simulink model "Copy_of_simulator"  (R2024a)
settings: Solver=VariableStepAuto  StartTime=0.0  StopTime=50  RelTol=1e-3
values from neighbouring files (symbols this model uses):
  g = inputs(6,1)    [measFunction.m]    (also in stateFunction.m)
  k_f = 6.11e-8    (= 6.11e-08)    [Data.m]
  k_m = 1.5e-9    (= 1.5e-09)    [Data.m]
undefined symbols (not defined in the file or in its folder): A, B, C, L, m
libraries: slpidlib x7, simulink x2, shared6dof x1, sharedutil x1
(part 1 of 2)
settings Model: Creator=matteocolussi  LastModifiedBy=matteocolussi

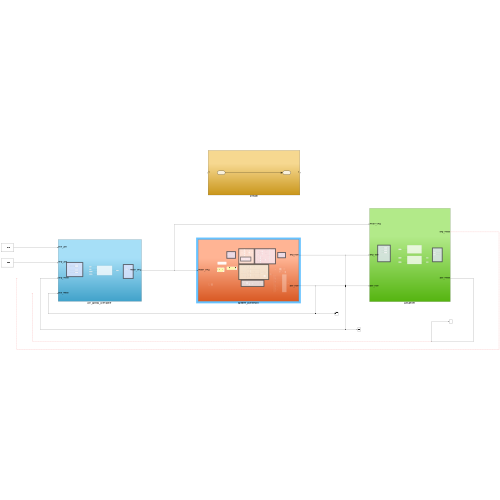
[thumbnail: Simulink's stored preview of the top-level diagram]
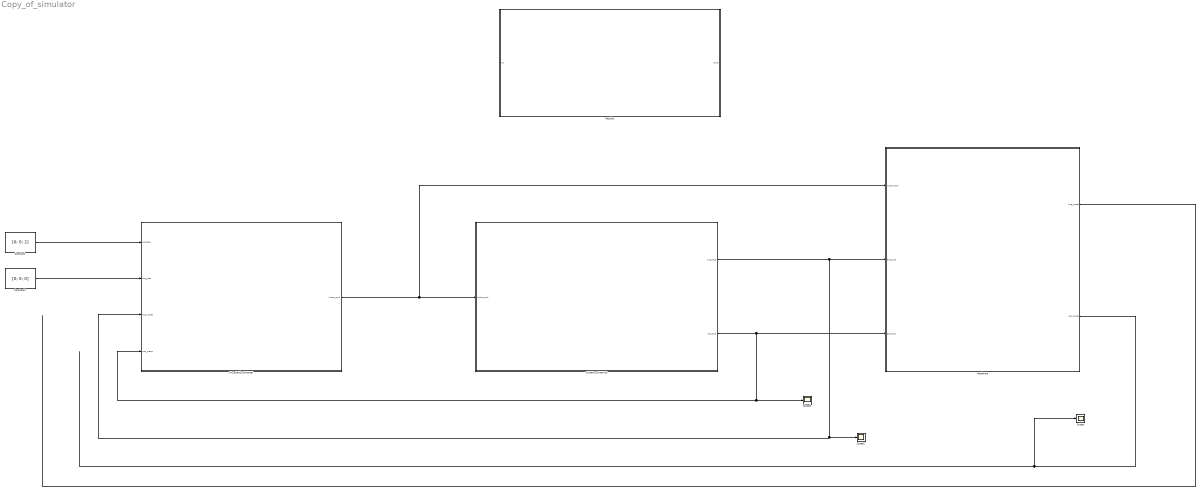
== system Copy_of_simulator ==
  Constant : Constant  Value=[0; 0; 2]
  Constant1 : Constant  Value=[0; 0; 0]
  Hardware : Subsystem
  On_Board_Computer : Subsystem
  Results : Subsystem
  Scope : Scope
  Scope1 : Scope
  Scope2 : Scope
  System_Dynamics : Subsystem
  wires:
  Constant1/1 -> On_Board_Computer/2(ang_des)
  On_Board_Computer/1(motor_cmd) -> Hardware/1(motor_cmd), System_Dynamics/1(motor_cmd)
  System_Dynamics/1(ang_true) -> Hardware/2(ang_true), On_Board_Computer/3(ang_meas), Scope2/1
  System_Dynamics/2(pos_true) -> Scope1/1, On_Board_Computer/4(pos_meas), Hardware/3(pos_true)
  Hardware/1(ang_meas) -> ?
  Hardware/2(pos_meas) -> Scope/1
  Constant/1 -> On_Board_Computer/1(pos_des)

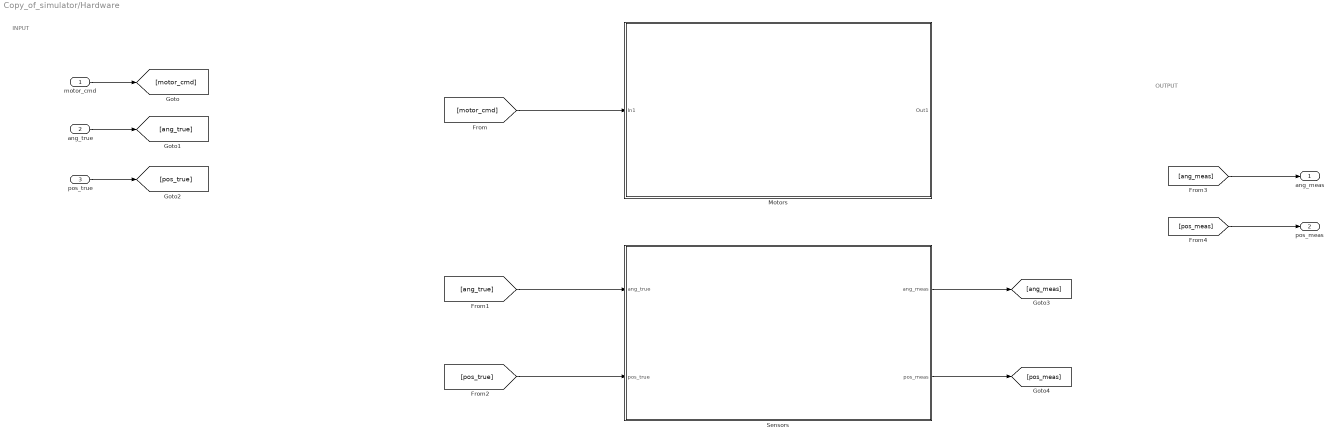
== system Copy_of_simulator/Hardware ==
  note: INPUT
  note: OUTPUT
  motor_cmd : Inport
  ang_true : Inport  Port=2
  pos_true : Inport  Port=3
  Motors : Subsystem
  Sensors : Subsystem
  ang_meas : Outport
  pos_meas : Outport  Port=2
  wires:
  motor_cmd/1 -> [motor_cmd]
  [motor_cmd] -> Motors/1(In1)
  ang_true/1 -> [ang_true]
  pos_true/1 -> [pos_true]
  [ang_true] -> Sensors/1(ang_true)
  [pos_true] -> Sensors/2(pos_true)
  Sensors/1(ang_meas) -> [ang_meas]
  Sensors/2(pos_meas) -> [pos_meas]
  [ang_meas] -> ang_meas/1
  [pos_meas] -> pos_meas/1

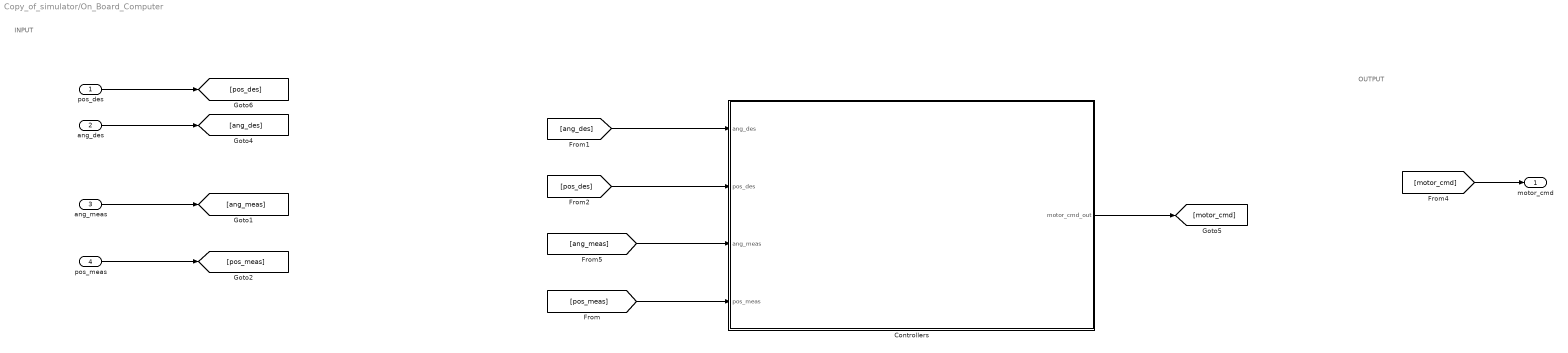
== system Copy_of_simulator/On_Board_Computer ==
  note: OUTPUT
  note: INPUT
  pos_des : Inport
  ang_des : Inport  Port=2
  ang_meas : Inport  Port=3
  pos_meas : Inport  Port=4
  Controllers : Subsystem
  motor_cmd : Outport
  wires:
  pos_des/1 -> [pos_des]
  [ang_des] -> Controllers/1(ang_des)
  [pos_des] -> Controllers/2(pos_des)
  ang_des/1 -> [ang_des]
  Controllers/1(motor_cmd_out) -> [motor_cmd]
  [motor_cmd] -> motor_cmd/1
  ang_meas/1 -> [ang_meas]
  pos_meas/1 -> [pos_meas]
  [pos_meas] -> Controllers/4(pos_meas)
  [ang_meas] -> Controllers/3(ang_meas)

== system Copy_of_simulator/Results ==
  In1 : Inport
  Out1 : Outport
  wires:
  In1/1 -> Out1/1

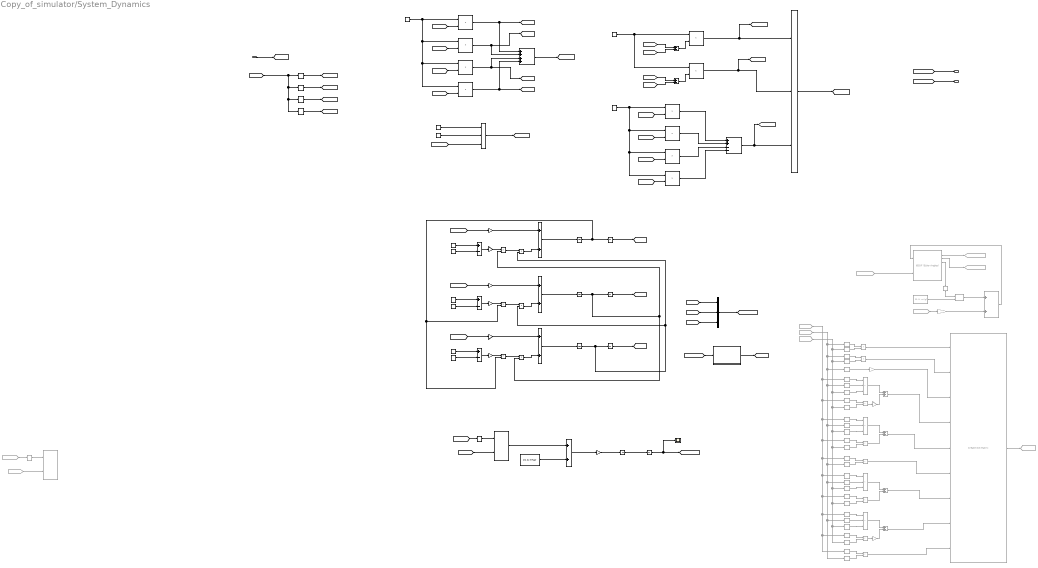
== system Copy_of_simulator/System_Dynamics ==
  note: ROTATIONAL DYNAMICS - EULER EQUATIONS
  note: FORCE VECTOR COMPUTATION
  note: Thrust computation
  note: INPUT
  note: Torque computation
  note: OUTPUT
  note: TRASLATIONAL DYNAMICS
  motor_cmd : Inport
  6DOF (Euler Angles) : shared6dof/6DOF (Euler Angles)  Commented=on  units=Metric (MKS)  mtype=Fixed  rep=Euler Angles  xme_0=[0 0 0]  Vm_0=[0 0 0]  eul_0=[0 0 0]  pm_0=[0 0 0]  mass_0=m  mass_e=0.5  mass_f=2.0  inertia=I  inertia_e=eye(3)  inertia_f=2*eye(3)  k_quat=1.0  vre_flag=on  abi_flag=on  aMode=0  xme_statename=''  Vm_statename=''  eul_statename=''  quat_statename=''  pm_statename=''  mass_statename=''
  Add{,1..4} (5 alike) : Sum  Inputs=+-
  Add{5,7..9} (4 alike) : Sum  Commented=on
  Add6 : Sum
  Constant : Constant  Value=k_f
  Constant1 : Constant  Value=k_m
  Constant10 : Constant  Value=A  VectorParams1D=off
  Constant11 : Constant  Value=B  VectorParams1D=off
  Constant13 : Constant  Value=[0, 0, m*g]'
  Constant14 : Constant  Commented=on  Value=[0; 0; -m*g]
  Constant2 : Constant  Value=L  VectorParams1D=off
  Constant3 : Constant  Value=0
  Constant4 : Constant  Value=0
  Constant5 : Constant  Value=C
  Constant6 : Constant  Value=B
  Constant7 : Constant  Value=C  VectorParams1D=off
  Constant9 : Constant  Value=A  VectorParams1D=off
  Cos{,1..4,6..8,12} (9 alike) : Trigonometry  Commented=on  Operator=cos
  Cos{5,9..11} (4 alike) : Trigonometry  Commented=on
  Create 3x3 Matrix : sharedutil/Create 3x3 Matrix  Commented=on  aMode=aMode
      settings: LibrarySourceBlock=aerolibutil/Create 3x3 Matrix
  From21 : From  Commented=on  GotoTag=F
  From23 : From  Commented=on  GotoTag=o_R_b
  From28 : From  Commented=on  GotoTag=F
  From29 : From  Commented=on  GotoTag=Mc
  From39 : From  Commented=on  GotoTag=phi_true
  From40 : From  Commented=on  GotoTag=theta_true
  From41 : From  Commented=on  GotoTag=psi_true
  Gain : Gain  Gain=1/A
  Gain1 : Gain  Gain=1/A
  Gain{6,8..10} (4 alike) : Gain  Commented=on  Gain=-1
  Gain2 : Gain  Gain=1/B
  Gain3 : Gain  Gain=1/B
  Gain4 : Gain  Gain=1/C
  Gain5 : Gain  Gain=1/C
  Gain7 : Gain  Gain=1/m
  Goto15 : Goto  Commented=on  GotoTag=o_R_b
  Goto29 : Goto  Commented=on  GotoTag=ang_true
  Goto30 : Goto  Commented=on  GotoTag=pos_true
  Integrator{6..11,18..19} (8 alike) : Integrator
  MATLAB Function : MATLAB Function  TreatAsAtomicUnit=on
  Matrix Multiply : Product  Commented=on  Multiplication=Matrix(*)
  Product{,1..9,11..16} (16 alike) : Product
  Product{10,19,21,23..24,26,28..29} (8 alike) : Product  Commented=on
  Product17 : Product  Commented=on  Multiplication=Matrix(*)
  Product18 : Product  Multiplication=Matrix(*)
  Product{20,22,25,27} (4 alike) : Product  Commented=on  Inputs=3
  Scope : Scope
  Selector : Selector  InputPortWidth=4  IndexOptions=Index vector (dialog)  Indices=1  OutputSizes=1
  Selector1 : Selector  InputPortWidth=4  IndexOptions=Index vector (dialog)  Indices=2  OutputSizes=1
  Selector2 : Selector  InputPortWidth=4  IndexOptions=Index vector (dialog)  Indices=3  OutputSizes=1
  Selector3 : Selector  InputPortWidth=4  IndexOptions=Index vector (dialog)  Indices=4  OutputSizes=1
  Sin{,1..6,8,10..11,13} (11 alike) : Trigonometry  Commented=on
  Sin{7,9,12,14..15} (5 alike) : Trigonometry  Commented=on  Operator=cos
  Sum : Sum  Inputs=++++
  Sum1 : Sum  Inputs=++--
  Sum2 : Sum
  Sum3 : Sum
  Sum4 : Sum
  Sum5 : Sum  Commented=on
  Transpose : Math  Commented=on  Operator=transpose
  Transpose1 : Math  Operator=transpose
  Transpose2 : Math  Commented=on  Operator=transpose
  Vector Concatenate : Concatenate  NumInputs=3
  Vector Concatenate1 : Concatenate  NumInputs=3
  Vector Concatenate3 : Concatenate  NumInputs=3
  ang_true : Outport
  pos_true : Outport  Port=2
  wires:
  motor_cmd/1 -> [motor_cmd]
  Selector/1 -> [w1_cmd]
  Selector1/1 -> [w2_cmd]
  Selector2/1 -> [w3_cmd]
  [motor_cmd] -> Selector3/1, Selector2/1, Selector1/1, Selector/1
  Selector3/1 -> [w4_cmd]
  Constant/1 -> Product3/1, Product2/1, Product1/1, Product/1
  [w1_cmd] -> Product/2
  [w2_cmd] -> Product1/2
  [w3_cmd] -> Product2/2
  [w4_cmd] -> Product3/2
  Product/1 -> [T1], Sum/1  "T1"
  Product1/1 -> Sum/2, [T2]  "T2"
  Product2/1 -> [T3], Sum/3  "T3"
  Product3/1 -> [T4], Sum/4  "T4"
  Sum/1 -> [T_tot]  "Thrust"
  [w2_cmd] -> Product5/2
  Constant1/1 -> Product7/1, Product6/1, Product5/1, Product4/1
  Product5/1 -> Sum1/2  "C2"
  Product6/1 -> Sum1/3  "C3"
  Product7/1 -> Sum1/4  "C4"
  [w1_cmd] -> Product4/2
  [w3_cmd] -> Product6/2
  Product4/1 -> Sum1/1  "C1"
  [w4_cmd] -> Product7/2
  Sum1/1 -> [Mc_zbody], Vector Concatenate/3  "Mc_zbody"
  Constant2/1 -> Product9/1, Product8/1
  [T3] -> Add/1
  [T4] -> Add/2
  Add/1 -> Product8/2
  [T2] -> Add1/1
  [T1] -> Add1/2
  Add1/1 -> Product9/2
  Product9/1 -> [Mc_ybody], Vector Concatenate/2  "Mc_ybody"
  Product8/1 -> [Mc_xbody], Vector Concatenate/1  "Mc_xbody"
  Vector Concatenate/1 -> [Mc]
  [T_tot] -> Vector Concatenate1/3
  Constant3/1 -> Vector Concatenate1/2
  Constant4/1 -> Vector Concatenate1/1
  Vector Concatenate1/1 -> [F]  "Force"
  [Mc_xbody] -> Gain1/1
  Constant6/1 -> Add2/1
  Add2/1 -> Gain/1
  Constant7/1 -> Add2/2
  Sum2/1 -> Integrator6/1  "phi_dotdot"
  Integrator7/1 -> [phi_true]  "phi"
  Gain/1 -> Product11/1
  Product11/1 -> Product12/1
  Product12/1 -> Sum2/2
  Gain1/1 -> Sum2/1
  Integrator9/1 -> [theta_true]  "theta"
  Gain3/1 -> Sum3/1
  Product14/1 -> Sum3/2
  [Mc_ybody] -> Gain3/1
  Gain2/1 -> Product13/1
  Integrator8/1 -> Integrator9/1, Product16/2, Product11/2  "theta_dot"
  Sum3/1 -> Integrator8/1  "theta_dotdot"
  Constant5/1 -> Add3/1
  Product13/1 -> Product14/1
  Add3/1 -> Gain2/1
  Constant9/1 -> Add3/2
  Integrator6/1 -> Integrator7/1, Product13/2, Product15/2  "phi_dot"
  Constant11/1 -> Add4/2
  Add4/1 -> Gain4/1
  Gain5/1 -> Sum4/1
  Constant10/1 -> Add4/1
  Gain4/1 -> Product15/1
  Integrator11/1 -> [psi_true]  "psi"
  Product16/1 -> Sum4/2
  [Mc_zbody] -> Gain5/1
  Integrator10/1 -> Product14/2, Product12/2, Integrator11/1  "psi_dot"
  Product15/1 -> Product16/1
  Sum4/1 -> Integrator10/1  "psi_dotdot"
  Vector Concatenate3/1 -> [ang_true]
  [theta_true] -> Vector Concatenate3/2
  [psi_true] -> Vector Concatenate3/3
  [phi_true] -> Vector Concatenate3/1
  From21/1 -> Transpose/1
  [ang_true] -> MATLAB Function/1(ang)
  MATLAB Function/1(o_R_b) -> [o_R_b]
  From23/1 -> Product17/2
  [ang_true] -> ang_true/1
  [pos_true] -> pos_true/1
  Transpose/1 -> Product17/1
  [F] -> Transpose1/1
  Add6/1 -> Gain7/1
  Transpose1/1 -> Product18/1
  Product18/1 -> Add6/1
  Gain7/1 -> Integrator18/1  "r_dotdot"
  [o_R_b] -> Product18/2
  Constant13/1 -> Add6/2
  Integrator18/1 -> Integrator19/1  "r_dot"
  Integrator19/1 -> [pos_true], Scope/1  "r"
  From29/1 -> 6DOF (Euler Angles)/2
  6DOF (Euler Angles)/3 -> Goto29/1
  6DOF (Euler Angles)/2 -> Goto30/1
  Constant14/1 -> Matrix Multiply/2
  6DOF (Euler Angles)/4 -> Transpose2/1
  From28/1 -> Gain8/1
  Matrix Multiply/1 -> Sum5/1
  Sum5/1 -> 6DOF (Euler Angles)/1
  Transpose2/1 -> Matrix Multiply/1
  Gain8/1 -> Sum5/2
  Cos/1 -> Product10/1
  Cos1/1 -> Product10/2
  Product10/1 -> Create 3x3 Matrix/1
  Product19/1 -> Create 3x3 Matrix/2
  Sin/1 -> Product19/2
  Cos2/1 -> Product19/1
  Sin1/1 -> Gain6/1
  Gain6/1 -> Create 3x3 Matrix/3
  Sin2/1 -> Product20/1
  Sin3/1 -> Product20/2
  Cos3/1 -> Product20/3
  Cos4/1 -> Product21/1
  Sin4/1 -> Product21/2
  Product20/1 -> Add5/1
  Product21/1 -> Gain9/1
  Gain9/1 -> Add5/2
  Add5/1 -> Create 3x3 Matrix/4
  Cos5/1 -> Product22/3
  Product22/1 -> Add7/1
  Add7/1 -> Create 3x3 Matrix/5
  Sin6/1 -> Product22/2
  Sin7/1 -> Product23/2
  Product23/1 -> Add7/2
  Sin5/1 -> Product22/1
  Cos6/1 -> Product23/1
  Sin8/1 -> Product24/1
  Cos7/1 -> Product24/2
  Product24/1 -> Create 3x3 Matrix/6
  Cos8/1 -> Product25/3
  Product25/1 -> Add8/1
  Sin11/1 -> Product26/2
  Add8/1 -> Create 3x3 Matrix/7
  Sin10/1 -> Product25/2
  Product26/1 -> Add8/2
  Sin9/1 -> Product25/1
  Cos9/1 -> Product26/1
  Product28/1 -> Gain10/1
  Cos10/1 -> Product27/3
  Product27/1 -> Add9/1
  Sin14/1 -> Product28/2
  Add9/1 -> Create 3x3 Matrix/8
  Sin13/1 -> Product27/2
  Gain10/1 -> Add9/2
  Sin12/1 -> Product27/1
  From41/1 -> Sin4/1, Cos5/1, Sin14/1, Cos10/1, Sin11/1, Cos8/1, Sin7/1, Cos3/1, Sin/1, Cos1/1
  Cos11/1 -> Product28/1
  Product29/1 -> Create 3x3 Matrix/9
  Sin15/1 -> Product29/2
  From39/1 -> Cos12/1, Cos11/1, Sin12/1, Cos9/1, Sin9/1, Sin8/1, Cos6/1, Sin5/1, Cos4/1, Sin2/1
  From40/1 -> Sin10/1, Sin15/1, Sin13/1, Cos7/1, Sin6/1, Sin3/1, Sin1/1, Cos2/1, Cos/1
  Cos12/1 -> Product29/1
  Create 3x3 Matrix/1 -> Goto15/1

== system Copy_of_simulator/Hardware/Motors ==
  In1 : Inport
  Out1 : Outport
  wires:
  In1/1 -> Out1/1

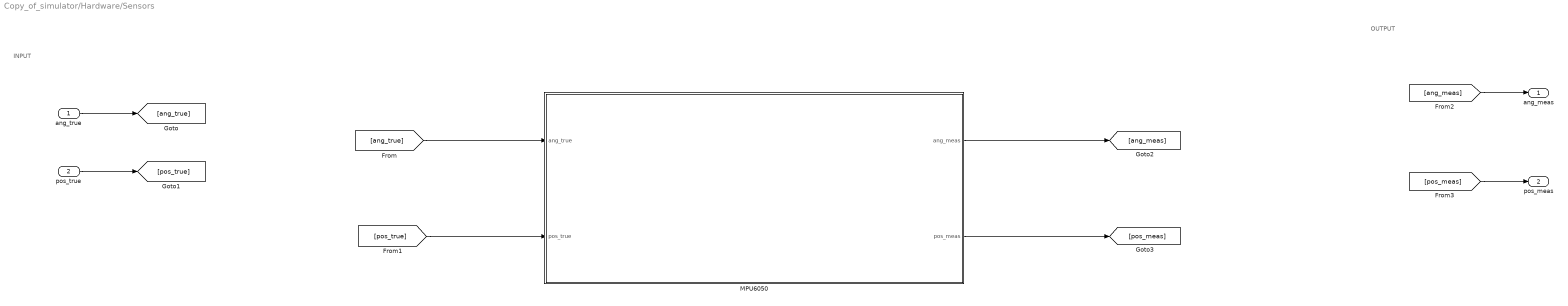
== system Copy_of_simulator/Hardware/Sensors ==
  note: OUTPUT
  note: INPUT
  ang_true : Inport
  pos_true : Inport  Port=2
  MPU6050 : Subsystem
  ang_meas : Outport
  pos_meas : Outport  Port=2
  wires:
  ang_true/1 -> [ang_true]
  pos_true/1 -> [pos_true]
  [ang_meas] -> ang_meas/1
  [pos_meas] -> pos_meas/1
  [ang_true] -> MPU6050/1(ang_true)
  [pos_true] -> MPU6050/2(pos_true)
  MPU6050/1(ang_meas) -> [ang_meas]
  MPU6050/2(pos_meas) -> [pos_meas]

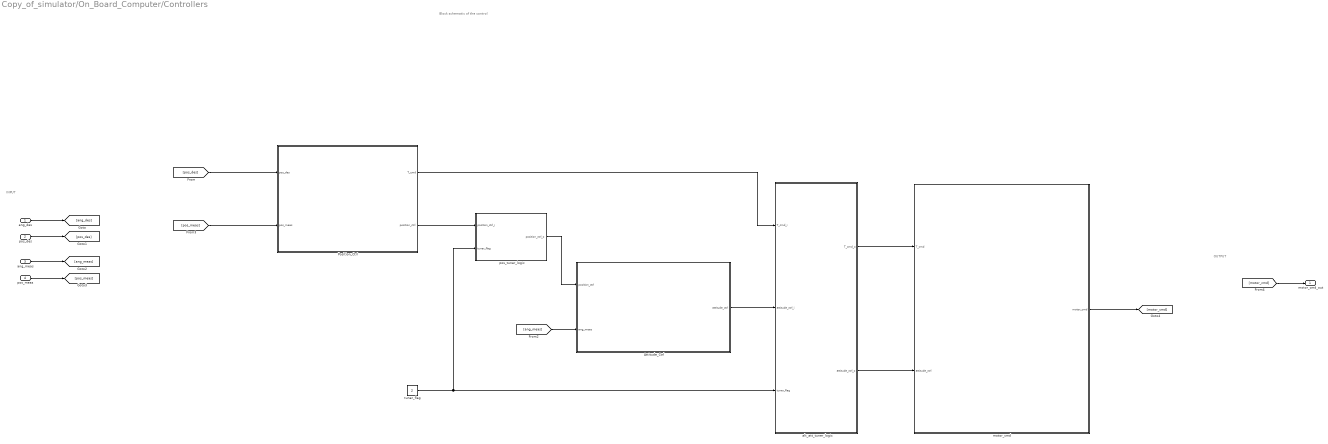
== system Copy_of_simulator/On_Board_Computer/Controllers ==
  note: Block schematic of the control
  note: OUTPUT
  note: INPUT
  ang_des : Inport
  pos_des : Inport  Port=2
  ang_meas : Inport  Port=3
  pos_meas : Inport  Port=4
  Attitude_Ctrl : Subsystem
  Position_Ctrl : Subsystem
  alt_att_tuner_logic : Subsystem
  motor_cmd : Subsystem
  pos_tuner_logic : Subsystem
  tuner_flag : Constant  Value=2
  motor_cmd_out : Outport
  wires:
  ang_des/1 -> [ang_des]
  pos_des/1 -> [pos_des]
  pos_meas/1 -> [pos_meas]
  ang_meas/1 -> [ang_meas]
  [ang_meas] -> Attitude_Ctrl/2(ang_meas)
  motor_cmd/1(motor_cmd) -> [motor_cmd]
  [motor_cmd] -> motor_cmd_out/1
  [pos_meas] -> Position_Ctrl/2(pos_meas)
  Attitude_Ctrl/1(attitude_ctrl) -> alt_att_tuner_logic/2(attitude_ctrl_i)
  tuner_flag/1 -> alt_att_tuner_logic/3(tuner_flag), pos_tuner_logic/2(tuner_flag)
  [pos_des] -> Position_Ctrl/1(pos_des)
  Position_Ctrl/2(position_ctrl) -> pos_tuner_logic/1(position_ctrl_i)
  pos_tuner_logic/1(position_ctrl_o) -> Attitude_Ctrl/1(position_ctrl)
  Position_Ctrl/1(T_cmd) -> alt_att_tuner_logic/1(T_cmd_i)
  alt_att_tuner_logic/1(T_cmd_o) -> motor_cmd/1(T_cmd)
  alt_att_tuner_logic/2(attitude_ctrl_o) -> motor_cmd/2(attitude_ctrl)

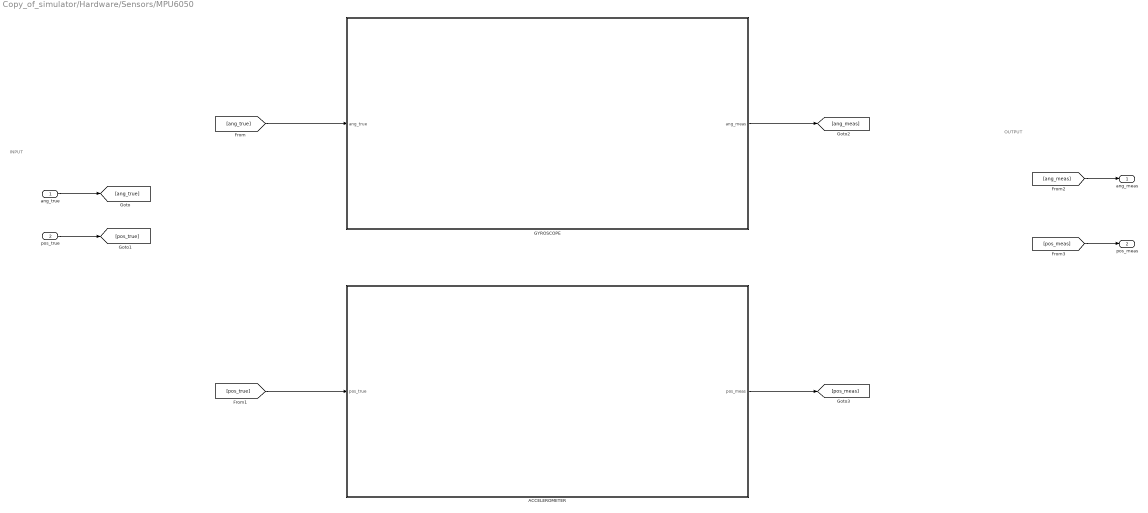
== system Copy_of_simulator/Hardware/Sensors/MPU6050 ==
  note: INPUT
  note: OUTPUT
  ang_true : Inport
  pos_true : Inport  Port=2
  ACCELEROMETER : Subsystem
  GYROSCOPE : Subsystem
  ang_meas : Outport
  pos_meas : Outport  Port=2
  wires:
  ang_true/1 -> [ang_true]
  pos_true/1 -> [pos_true]
  [pos_meas] -> pos_meas/1
  [ang_meas] -> ang_meas/1
  [ang_true] -> GYROSCOPE/1(ang_true)
  [pos_true] -> ACCELEROMETER/1(pos_true)
  GYROSCOPE/1(ang_meas) -> [ang_meas]
  ACCELEROMETER/1(pos_meas) -> [pos_meas]

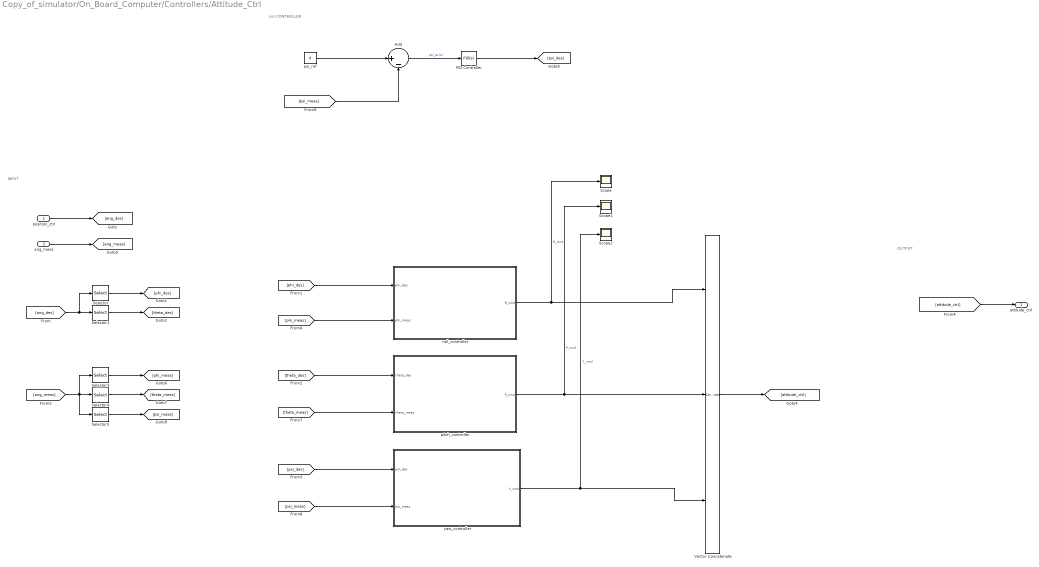
== system Copy_of_simulator/On_Board_Computer/Controllers/Attitude_Ctrl ==
  note: OUTPUT
  note: INPUT
  note: psi CONTROLLER
  position_ctrl : Inport
  ang_meas : Inport  Port=2
  Add : Sum  Inputs=|+-
  PID Controller : slpidlib/PID Controller  Controller=PID  Form=Parallel  TimeDomain=Continuous-time  UseExternalTs=off  SampleTime=-1  IntegratorMethod=Forward Euler  FilterMethod=Forward Euler  ControllerParametersSource=internal  P=1  I=0.8  UseKiTs=off  D=0.2  UseExternalDerivativeSource=off  N=100  UseFilter=on  TunerSelectOption=Transfer Function Based (PID Tuner App)  InitialConditionSource=internal  InitialConditionForIntegrator=0  InitialConditionForFilter=0  DifferentiatorICPrevScaledInput=0  ExternalReset=none  TrackingMode=off  Kt=1  LimitOutput=off  SatLimitsSource=internal  UpperSaturationLimit=inf  LowerSaturationLimit=-inf  LinearizeAsGain=on  AntiWindupMode=none  Kb=1  LimitIntegrator=off  UpperIntegratorSaturationLimit=inf  LowerIntegratorSaturationLimit=-inf  POutMin=[]  POutMax=[]  IOutMin=[]  IOutMax=[]  DOutMin=[]  DOutMax=[]  NOutMin=[]  NOutMax=[]  SumOutMin=[]  SumOutMax=[]  SaturationOutMin=[]  SaturationOutMax=[]  PParamMin=[]  PParamMax=[]  IParamMin=[]  IParamMax=[]  DParamMin=[]  DParamMax=[]  NParamMin=[]  NParamMax=[]  KbParamMin=[]  KbParamMax=[]  KtParamMin=[]  KtParamMax=[]  KbOutMin=[]  KbOutMax=[]  KtOutMin=[]  KtOutMax=[]  IntegratorOutMin=[]  IntegratorOutMax=[]  FilterOutMin=[]  FilterOutMax=[]  SumI1OutMin=[]  SumI1OutMax=[]  SumI2OutMin=[]  SumI2OutMax=[]  SumI3OutMin=[]  SumI3OutMax=[]  SumI4OutMin=[]  SumI4OutMax=[]  SumDOutMin=[]  SumDOutMax=[]  DifferentiatorOutMin=[]  DifferentiatorOutMax=[]  FilterDiffOutCoefMin=[]  FilterDiffOutCoefMax=[]  ReciprocalOutMin=[]  ReciprocalOutMax=[]  SumDenOutMin=[]  SumDenOutMax=[]  SumNumOutMin=[]  SumNumOutMax=[]  DivideOutMin=[]  DivideOutMax=[]  UdiffTsProdOutMin=[]  UdiffTsProdOutMax=[]  NTsProdOutMin=[]  NTsProdOutMax=[]  UintegralTsProdOutMin=[]  UintegralTsProdOutMax=[]  UngainTsProdOutMin=[]  UngainTsProdOutMax=[]  ClampingZeroOutDataTypeStr=Inherit: Inherit via back propagation  ClampingZeroOutMin=[]  ClampingZeroOutMax=[]  FilterDenConstantOutDataTypeStr=Inherit: Inherit via back propagation  FilterDenConstantOutMin=[]  FilterDenConstantOutMax=[]  PCopyOutDataTypeStr=Inherit: Inherit via back propagation  PCopyOutMin=[]  PCopyOutMax=[]  NCopyOutDataTypeStr=Inherit: Inherit via back propagation  NCopyOutMin=[]  NCopyOutMax=[]  IntegratorContinuousStateAttributes=''  IntegratorStateMustResolveToSignalObject=off  IntegratorRTWStateStorageClass=Auto  FilterContinuousStateAttributes=''  FilterStateMustResolveToSignalObject=off  FilterRTWStateStorageClass=Auto  ParallelPVariant=InternalParameters  IdealPVariant=Disabled  IVariant=InternalParameters  DVariant=InternalParameters  IntegratorVariant=Continuous  SatVariant=Disabled  AWVariant=Passthrough  PCopyVariant=Disabled  TRVariant=Disabled  FdbkBlocksVariant=Forward  IdealPFdbkVariant=Disabled  SatFdbkVariant=Disabled  DerivativeFilterVariant=ContFilter  NVariant=InternalParameters  NCopyVariant=Disabled  FilterICVariant=InternalICsFilter  IntegratorICVariant=InternalICs  ExternalResetVariant=Disabled  TRSumVariant=Passthrough  SumFdbkVariant=Disabled  SumVariant=Sum_PID  TsampFilterVariant=InternalTs  TsampNgainVariant=Passthrough  TsampIntegralVariant=Disabled_SignalSpec  ExternalSaturationOutDataTypeStr=Inherit: Same as second input  DerivativeSourceVariant=ErrorSignal
  Scope : Scope
  Scope1 : Scope
  Scope2 : Scope
  Selector : Selector  InputPortWidth=2  IndexOptions=Index vector (dialog)  Indices=1  OutputSizes=1
  Selector1 : Selector  InputPortWidth=2  IndexOptions=Index vector (dialog)  Indices=2  OutputSizes=1
  Selector3 : Selector  InputPortWidth=3  IndexOptions=Index vector (dialog)  Indices=1  OutputSizes=1
  Selector4 : Selector  InputPortWidth=3  IndexOptions=Index vector (dialog)  Indices=2  OutputSizes=1
  Selector5 : Selector  InputPortWidth=3  IndexOptions=Index vector (dialog)  Indices=3  OutputSizes=1
  Vector Concatenate : Concatenate  NumInputs=3
  pitch_controller : Subsystem
  psi_ref : Constant  Value=0
  roll_controller : Subsystem
  yaw_controller : Subsystem
  attitude_ctrl : Outport
  wires:
  position_ctrl/1 -> [ang_des]
  [phi_des] -> roll_controller/1(phi_des)
  [theta_des] -> pitch_controller/1(theta_des)
  [psi_des] -> yaw_controller/1(psi_des)
  roll_controller/1(R_cmd) -> Vector Concatenate/1, Scope/1  "R_cmd"
  pitch_controller/1(P_cmd) -> Scope1/1, Vector Concatenate/2  "P_cmd"
  yaw_controller/1(Y_cmd) -> Scope2/1, Vector Concatenate/3  "Y_cmd"
  ang_meas/1 -> [ang_meas]
  [phi_meas] -> roll_controller/2(phi_meas)
  [theta_meas] -> pitch_controller/2(theta_meas)
  [psi_meas] -> yaw_controller/2(psi_meas)
  Selector/1 -> [phi_des]
  [ang_des] -> Selector1/1, Selector/1
  Selector1/1 -> [theta_des]
  [ang_meas] -> Selector5/1, Selector4/1, Selector3/1
  Selector4/1 -> [theta_meas]
  Selector5/1 -> [psi_meas]
  Selector3/1 -> [phi_meas]
  Vector Concatenate/1 -> [attitude_ctrl]
  [attitude_ctrl] -> attitude_ctrl/1
  psi_ref/1 -> Add/1
  Add/1 -> PID Controller/1  "psi_error"
  PID Controller/1 -> [psi_des]
  [psi_meas] -> Add/2

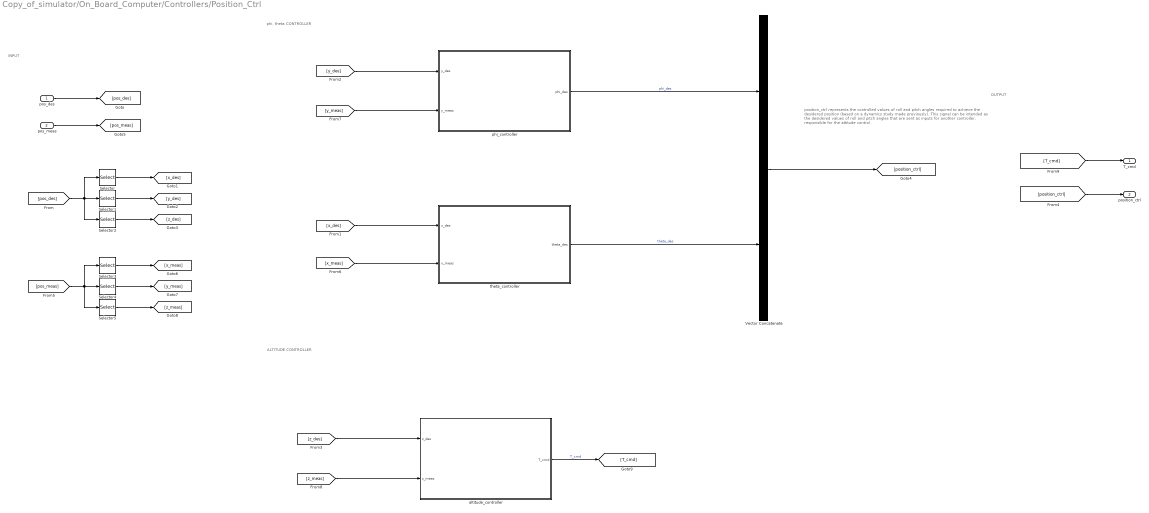
== system Copy_of_simulator/On_Board_Computer/Controllers/Position_Ctrl ==
  note: position_ctrl represents the controlled values of roll and pitch angles required to achieve the desidered position (based on a dynamics study made previously).
      |
      | This signal can be intended as the desidered values of roll and pitch angles that are sent as inputs for another controller, responsible for the attitude control .
  note: ALTITUDE CONTROLLER
  note: phi, theta CONTROLLER
  note: INPUT
  note: OUTPUT
  pos_des : Inport
  pos_meas : Inport  Port=2
  Selector : Selector  InputPortWidth=3  IndexOptions=Index vector (dialog)  Indices=1  OutputSizes=1
  Selector1 : Selector  InputPortWidth=3  IndexOptions=Index vector (dialog)  Indices=2  OutputSizes=1
  Selector2 : Selector  InputPortWidth=3  IndexOptions=Index vector (dialog)  Indices=3  OutputSizes=1
  Selector3 : Selector  InputPortWidth=3  IndexOptions=Index vector (dialog)  Indices=1  OutputSizes=1
  Selector4 : Selector  InputPortWidth=3  IndexOptions=Index vector (dialog)  Indices=2  OutputSizes=1
  Selector5 : Selector  InputPortWidth=3  IndexOptions=Index vector (dialog)  Indices=3  OutputSizes=1
  Vector Concatenate : Concatenate
  altitude_controller : Subsystem
  phi_controller : Subsystem
  theta_controller : Subsystem
  T_cmd : Outport
  position_ctrl : Outport  Port=2
  wires:
  Selector3/1 -> [x_meas]
  Selector4/1 -> [y_meas]
  [pos_meas] -> Selector5/1, Selector4/1, Selector3/1
  pos_meas/1 -> [pos_meas]
  Selector5/1 -> [z_meas]
  [pos_des] -> Selector2/1, Selector1/1, Selector/1
  Selector/1 -> [x_des]
  pos_des/1 -> [pos_des]
  Selector1/1 -> [y_des]
  Selector2/1 -> [z_des]
  [y_meas] -> phi_controller/2(y_meas)
  [x_des] -> theta_controller/1(x_des)
  [y_des] -> phi_controller/1(y_des)
  [x_meas] -> theta_controller/2(x_meas)
  [position_ctrl] -> position_ctrl/1
  Vector Concatenate/1 -> [position_ctrl]
  theta_controller/1(theta_des) -> Vector Concatenate/2  "theta_des"
  [z_meas] -> altitude_controller/2(z_meas)
  [z_des] -> altitude_controller/1(z_des)
  altitude_controller/1(T_cmd) -> [T_cmd]  "T_cmd"
  [T_cmd] -> T_cmd/1
  phi_controller/1(phi_des) -> Vector Concatenate/1  "phi_des"

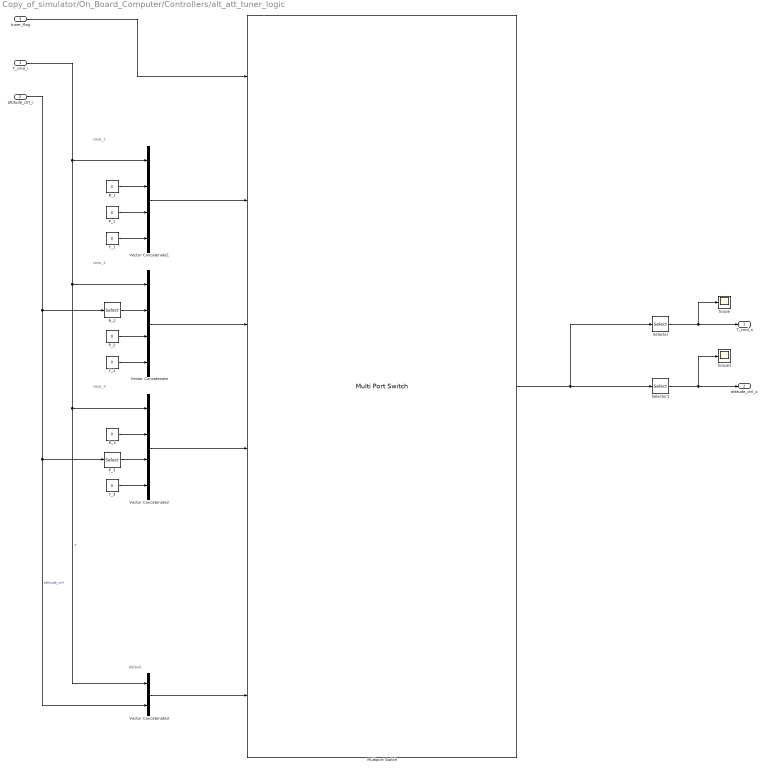
== system Copy_of_simulator/On_Board_Computer/Controllers/alt_att_tuner_logic ==
  note: case_2
  note: case_1
  note: case_3
  note: default
  T_cmd_i : Inport
  attitude_ctrl_i : Inport  Port=2
  tuner_flag : Inport  Port=3
  Multiport Switch : MultiPortSwitch  Inputs=5  SaturateOnIntegerOverflow=off  InputSameDT=off
  P_1 : Constant  Value=0
  P_2 : Constant  Value=0
  P_3 : Selector  InputPortWidth=3  IndexOptions=Index vector (dialog)  Indices=2  OutputSizes=1
  R_1 : Constant  Value=0
  R_2 : Selector  InputPortWidth=3  IndexOptions=Index vector (dialog)  Indices=1  OutputSizes=1
  R_3 : Constant  Value=0
  Scope : Scope
  Scope1 : Scope
  Selector : Selector  InputPortWidth=4  IndexOptions=Index vector (dialog)  Indices=1  OutputSizes=1
  Selector1 : Selector  InputPortWidth=4  IndexOptions=Index vector (dialog)  Indices=2:4  OutputSizes=1
  Vector Concatenate : Concatenate  NumInputs=4
  Vector Concatenate1 : Concatenate  NumInputs=4
  Vector Concatenate2 : Concatenate  NumInputs=4
  Vector Concatenate3 : Concatenate
  Y_1 : Constant  Value=0
  Y_2 : Constant  Value=0
  Y_3 : Constant  Value=0
  T_cmd_o : Outport
  attitude_ctrl_o : Outport  Port=2
  wires:
  tuner_flag/1 -> Multiport Switch/1
  Vector Concatenate/1 -> Multiport Switch/3
  P_2/1 -> Vector Concatenate/3
  Y_2/1 -> Vector Concatenate/4
  Multiport Switch/1 -> Selector/1, Selector1/1
  Selector/1 -> Scope/1, T_cmd_o/1
  Selector1/1 -> Scope1/1, attitude_ctrl_o/1
  R_2/1 -> Vector Concatenate/2
  R_1/1 -> Vector Concatenate1/2
  P_1/1 -> Vector Concatenate1/3
  Y_1/1 -> Vector Concatenate1/4
  Vector Concatenate1/1 -> Multiport Switch/2
  P_3/1 -> Vector Concatenate2/3
  Y_3/1 -> Vector Concatenate2/4
  Vector Concatenate2/1 -> Multiport Switch/4
  R_3/1 -> Vector Concatenate2/2
  T_cmd_i/1 -> Vector Concatenate3/1, Vector Concatenate2/1, Vector Concatenate/1, Vector Concatenate1/1  "T"
  Vector Concatenate3/1 -> Multiport Switch/6
  attitude_ctrl_i/1 -> Vector Concatenate3/2, P_3/1, R_2/1  "attitude_ctrl"

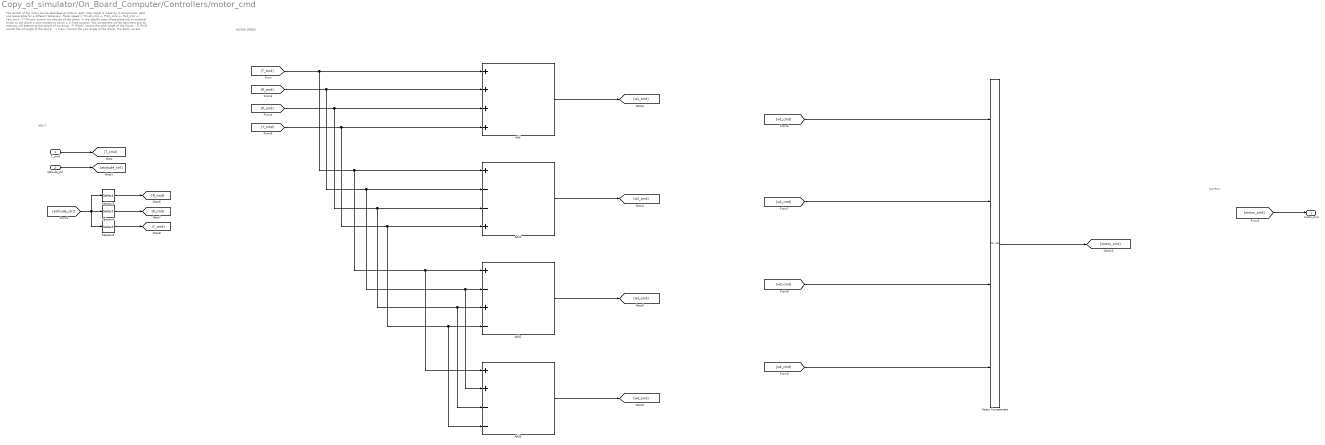
== system Copy_of_simulator/On_Board_Computer/Controllers/motor_cmd ==
  note: The control of the rotors can be described as follows:
      |
      | each rotor signal is made by 4 components, each one responsible for a different behaviour:
      |
      | Rotor speed = Thrust_cmd +- Pitch_cmd +- Roll_cmd +- Yaw_cmd
      |
      | - T (Thrust): control the altitude of the drone. In the specific case where there are no
      | external forces or the drone is commanded to hover in a fixed position,
      | this component will be dominant and its intensity will determine the height
      | of hovering;
      | - P (Pitch): control the pitch angle of the drone;
      | - R (Roll): control the roll angle of the drone;
      | - Y (Yaw): control the yaw angle of the drone;
      |
      | The block we are currently in is responsible for the computation of each component and their correct combination, which is different for every single rotor.
  note: MOTOR SPEED
  note: OUTPUT
  note: INPUT
  T_cmd : Inport
  attitude_ctrl : Inport  Port=2
  Add : Sum  Inputs=++++
  Add1 : Sum  Inputs=+--+
  Add2 : Sum  Inputs=+-+-
  Add3 : Sum  Inputs=++--
  Selector3 : Selector  InputPortWidth=3  IndexOptions=Index vector (dialog)  Indices=1  OutputSizes=1
  Selector4 : Selector  InputPortWidth=3  IndexOptions=Index vector (dialog)  Indices=2  OutputSizes=1
  Selector5 : Selector  InputPortWidth=3  IndexOptions=Index vector (dialog)  Indices=3  OutputSizes=1
  Vector Concatenate : Concatenate  NumInputs=4
  motor_cmd : Outport
  wires:
  T_cmd/1 -> [T_cmd]
  [motor_cmd] -> motor_cmd/1
  attitude_ctrl/1 -> [attitude_ctrl]
  Selector3/1 -> [R_cmd]
  Selector4/1 -> [P_cmd]
  [attitude_ctrl] -> Selector5/1, Selector4/1, Selector3/1
  Selector5/1 -> [Y_cmd]
  [T_cmd] -> Add/1, Add2/1, Add3/1, Add1/1
  [R_cmd] -> Add/2, Add3/2, Add2/2, Add1/2
  [P_cmd] -> Add/3, Add1/3, Add3/3, Add2/3
  [Y_cmd] -> Add/4, Add1/4, Add3/4, Add2/4
  Add/1 -> [w1_cmd]
  Add1/1 -> [w2_cmd]
  Add2/1 -> [w3_cmd]
  Add3/1 -> [w4_cmd]
  Vector Concatenate/1 -> [motor_cmd]
  [w2_cmd] -> Vector Concatenate/2
  [w1_cmd] -> Vector Concatenate/1
  [w3_cmd] -> Vector Concatenate/3
  [w4_cmd] -> Vector Concatenate/4

== system Copy_of_simulator/On_Board_Computer/Controllers/pos_tuner_logic ==
  note: case_2
  note: case_3
  position_ctrl_i : Inport
  tuner_flag : Inport  Port=2
  Multiport Switch : MultiPortSwitch  Inputs=5  SaturateOnIntegerOverflow=off  InputSameDT=off
  Scope : Scope
  Vector Concatenate : Concatenate
  Vector Concatenate1 : Concatenate
  phi_des_2 : Constant  Value=2
  phi_des_3 : Constant  Value=0
  theta_des_2 : Constant  Value=0
  theta_des_3 : Constant  Value=2
  position_ctrl_o : Outport
  wires:
  tuner_flag/1 -> Multiport Switch/1
  Multiport Switch/1 -> Scope/1, position_ctrl_o/1
  position_ctrl_i/1 -> Multiport Switch/6
  Vector Concatenate/1 -> Multiport Switch/3
  phi_des_2/1 -> Vector Concatenate/1
  theta_des_2/1 -> Vector Concatenate/2
  theta_des_3/1 -> Vector Concatenate1/2
  phi_des_3/1 -> Vector Concatenate1/1
  Vector Concatenate1/1 -> Multiport Switch/4

== system Copy_of_simulator/Hardware/Sensors/MPU6050/ACCELEROMETER ==
  pos_true : Inport
  Band-Limited White Noise : simulink/Sources/Band-Limited White Noise  Cov=[0.1]  Ts=0.1  seed=[23341]
  Sum : Sum  Inputs=|++
  pos_meas : Outport
  wires:
  Band-Limited White Noise/1 -> Sum/2
  pos_true/1 -> Sum/1
  Sum/1 -> pos_meas/1

== system Copy_of_simulator/Hardware/Sensors/MPU6050/GYROSCOPE ==
  ang_true : Inport
  Band-Limited White Noise : simulink/Sources/Band-Limited White Noise  Cov=[0.1]  Ts=0.1  seed=[23341]
  Sum : Sum  Inputs=|++
  ang_meas : Outport
  wires:
  ang_true/1 -> Sum/1
  Band-Limited White Noise/1 -> Sum/2
  Sum/1 -> ang_meas/1

== system Copy_of_simulator/On_Board_Computer/Controllers/Attitude_Ctrl/pitch_controller ==
  note: OUTPUT
  note: INPUT
  note: SENSOR DYNAMICS
      | TBD
  theta_des : Inport
  theta_meas : Inport  Port=2
  Add : Sum  Inputs=|+-
  PID Controller : slpidlib/PID Controller  Controller=PID  Form=Parallel  TimeDomain=Continuous-time  UseExternalTs=off  SampleTime=-1  IntegratorMethod=Forward Euler  FilterMethod=Forward Euler  ControllerParametersSource=internal  P=-17625.8547786025  I=-825.150483451763  UseKiTs=off  D=-92450.7642106306  UseExternalDerivativeSource=off  N=5.45397025421619  UseFilter=on  TunerSelectOption=Transfer Function Based (PID Tuner App)  InitialConditionSource=internal  InitialConditionForIntegrator=0  InitialConditionForFilter=0  DifferentiatorICPrevScaledInput=0  ExternalReset=none  TrackingMode=off  Kt=1  LimitOutput=off  SatLimitsSource=internal  UpperSaturationLimit=inf  LowerSaturationLimit=-inf  LinearizeAsGain=on  AntiWindupMode=none  Kb=1  LimitIntegrator=off  UpperIntegratorSaturationLimit=inf  LowerIntegratorSaturationLimit=-inf  POutMin=[]  POutMax=[]  IOutMin=[]  IOutMax=[]  DOutMin=[]  DOutMax=[]  NOutMin=[]  NOutMax=[]  SumOutMin=[]  SumOutMax=[]  SaturationOutMin=[]  SaturationOutMax=[]  PParamMin=[]  PParamMax=[]  IParamMin=[]  IParamMax=[]  DParamMin=[]  DParamMax=[]  NParamMin=[]  NParamMax=[]  KbParamMin=[]  KbParamMax=[]  KtParamMin=[]  KtParamMax=[]  KbOutMin=[]  KbOutMax=[]  KtOutMin=[]  KtOutMax=[]  IntegratorOutMin=[]  IntegratorOutMax=[]  FilterOutMin=[]  FilterOutMax=[]  SumI1OutMin=[]  SumI1OutMax=[]  SumI2OutMin=[]  SumI2OutMax=[]  SumI3OutMin=[]  SumI3OutMax=[]  SumI4OutMin=[]  SumI4OutMax=[]  SumDOutMin=[]  SumDOutMax=[]  DifferentiatorOutMin=[]  DifferentiatorOutMax=[]  FilterDiffOutCoefMin=[]  FilterDiffOutCoefMax=[]  ReciprocalOutMin=[]  ReciprocalOutMax=[]  SumDenOutMin=[]  SumDenOutMax=[]  SumNumOutMin=[]  SumNumOutMax=[]  DivideOutMin=[]  DivideOutMax=[]  UdiffTsProdOutMin=[]  UdiffTsProdOutMax=[]  NTsProdOutMin=[]  NTsProdOutMax=[]  UintegralTsProdOutMin=[]  UintegralTsProdOutMax=[]  UngainTsProdOutMin=[]  UngainTsProdOutMax=[]  ClampingZeroOutDataTypeStr=Inherit: Inherit via back propagation  ClampingZeroOutMin=[]  ClampingZeroOutMax=[]  FilterDenConstantOutDataTypeStr=Inherit: Inherit via back propagation  FilterDenConstantOutMin=[]  FilterDenConstantOutMax=[]  PCopyOutDataTypeStr=Inherit: Inherit via back propagation  PCopyOutMin=[]  PCopyOutMax=[]  NCopyOutDataTypeStr=Inherit: Inherit via back propagation  NCopyOutMin=[]  NCopyOutMax=[]  IntegratorContinuousStateAttributes=''  IntegratorStateMustResolveToSignalObject=off  IntegratorRTWStateStorageClass=Auto  FilterContinuousStateAttributes=''  FilterStateMustResolveToSignalObject=off  FilterRTWStateStorageClass=Auto  ParallelPVariant=InternalParameters  IdealPVariant=Disabled  IVariant=InternalParameters  DVariant=InternalParameters  IntegratorVariant=Continuous  SatVariant=Disabled  AWVariant=Passthrough  PCopyVariant=Disabled  TRVariant=Disabled  FdbkBlocksVariant=Forward  IdealPFdbkVariant=Disabled  SatFdbkVariant=Disabled  DerivativeFilterVariant=ContFilter  NVariant=InternalParameters  NCopyVariant=Disabled  FilterICVariant=InternalICsFilter  IntegratorICVariant=InternalICs  ExternalResetVariant=Disabled  TRSumVariant=Passthrough  SumFdbkVariant=Disabled  SumVariant=Sum_PID  TsampFilterVariant=InternalTs  TsampNgainVariant=Passthrough  TsampIntegralVariant=Disabled_SignalSpec  ExternalSaturationOutDataTypeStr=Inherit: Same as second input  DerivativeSourceVariant=ErrorSignal
  P_cmd : Outport
  wires:
  Add/1 -> PID Controller/1  "theta_error"
  [P_cmd] -> P_cmd/1
  [theta_des] -> Add/1
  theta_des/1 -> [theta_des]
  PID Controller/1 -> [P_cmd]
  theta_meas/1 -> [theta_meas]
  [theta_meas] -> Add/2

== system Copy_of_simulator/On_Board_Computer/Controllers/Attitude_Ctrl/roll_controller ==
  note: OUTPUT
  note: INPUT
  phi_des : Inport
  phi_meas : Inport  Port=2
  Add : Sum  Inputs=|+-
  PID Controller : slpidlib/PID Controller  Controller=PID  Form=Parallel  TimeDomain=Continuous-time  UseExternalTs=off  SampleTime=-1  IntegratorMethod=Forward Euler  FilterMethod=Forward Euler  ControllerParametersSource=internal  P=-17625.8547786025  I=-825.150483451763  UseKiTs=off  D=-92450.7642106305  UseExternalDerivativeSource=off  N=5.45397025421619  UseFilter=on  TunerSelectOption=Transfer Function Based (PID Tuner App)  InitialConditionSource=internal  InitialConditionForIntegrator=0  InitialConditionForFilter=0  DifferentiatorICPrevScaledInput=0  ExternalReset=none  TrackingMode=off  Kt=1  LimitOutput=off  SatLimitsSource=internal  UpperSaturationLimit=inf  LowerSaturationLimit=-inf  LinearizeAsGain=on  AntiWindupMode=none  Kb=1  LimitIntegrator=off  UpperIntegratorSaturationLimit=inf  LowerIntegratorSaturationLimit=-inf  POutMin=[]  POutMax=[]  IOutMin=[]  IOutMax=[]  DOutMin=[]  DOutMax=[]  NOutMin=[]  NOutMax=[]  SumOutMin=[]  SumOutMax=[]  SaturationOutMin=[]  SaturationOutMax=[]  PParamMin=[]  PParamMax=[]  IParamMin=[]  IParamMax=[]  DParamMin=[]  DParamMax=[]  NParamMin=[]  NParamMax=[]  KbParamMin=[]  KbParamMax=[]  KtParamMin=[]  KtParamMax=[]  KbOutMin=[]  KbOutMax=[]  KtOutMin=[]  KtOutMax=[]  IntegratorOutMin=[]  IntegratorOutMax=[]  FilterOutMin=[]  FilterOutMax=[]  SumI1OutMin=[]  SumI1OutMax=[]  SumI2OutMin=[]  SumI2OutMax=[]  SumI3OutMin=[]  SumI3OutMax=[]  SumI4OutMin=[]  SumI4OutMax=[]  SumDOutMin=[]  SumDOutMax=[]  DifferentiatorOutMin=[]  DifferentiatorOutMax=[]  FilterDiffOutCoefMin=[]  FilterDiffOutCoefMax=[]  ReciprocalOutMin=[]  ReciprocalOutMax=[]  SumDenOutMin=[]  SumDenOutMax=[]  SumNumOutMin=[]  SumNumOutMax=[]  DivideOutMin=[]  DivideOutMax=[]  UdiffTsProdOutMin=[]  UdiffTsProdOutMax=[]  NTsProdOutMin=[]  NTsProdOutMax=[]  UintegralTsProdOutMin=[]  UintegralTsProdOutMax=[]  UngainTsProdOutMin=[]  UngainTsProdOutMax=[]  ClampingZeroOutDataTypeStr=Inherit: Inherit via back propagation  ClampingZeroOutMin=[]  ClampingZeroOutMax=[]  FilterDenConstantOutDataTypeStr=Inherit: Inherit via back propagation  FilterDenConstantOutMin=[]  FilterDenConstantOutMax=[]  PCopyOutDataTypeStr=Inherit: Inherit via back propagation  PCopyOutMin=[]  PCopyOutMax=[]  NCopyOutDataTypeStr=Inherit: Inherit via back propagation  NCopyOutMin=[]  NCopyOutMax=[]  IntegratorContinuousStateAttributes=''  IntegratorStateMustResolveToSignalObject=off  IntegratorRTWStateStorageClass=Auto  FilterContinuousStateAttributes=''  FilterStateMustResolveToSignalObject=off  FilterRTWStateStorageClass=Auto  ParallelPVariant=InternalParameters  IdealPVariant=Disabled  IVariant=InternalParameters  DVariant=InternalParameters  IntegratorVariant=Continuous  SatVariant=Disabled  AWVariant=Passthrough  PCopyVariant=Disabled  TRVariant=Disabled  FdbkBlocksVariant=Forward  IdealPFdbkVariant=Disabled  SatFdbkVariant=Disabled  DerivativeFilterVariant=ContFilter  NVariant=InternalParameters  NCopyVariant=Disabled  FilterICVariant=InternalICsFilter  IntegratorICVariant=InternalICs  ExternalResetVariant=Disabled  TRSumVariant=Passthrough  SumFdbkVariant=Disabled  SumVariant=Sum_PID  TsampFilterVariant=InternalTs  TsampNgainVariant=Passthrough  TsampIntegralVariant=Disabled_SignalSpec  ExternalSaturationOutDataTypeStr=Inherit: Same as second input  DerivativeSourceVariant=ErrorSignal
  R_cmd : Outport
  wires:
  phi_des/1 -> [phi_des]
  [phi_des] -> Add/1
  [R_cmd] -> R_cmd/1
  phi_meas/1 -> [phi_meas]
  [phi_meas] -> Add/2
  Add/1 -> PID Controller/1  "phi_error"
  PID Controller/1 -> [R_cmd]

== system Copy_of_simulator/On_Board_Computer/Controllers/Attitude_Ctrl/yaw_controller ==
  note: OUTPUT
  note: INPUT
  note: SENSOR DYNAMICS
      | TBD
  psi_des : Inport
  psi_meas : Inport  Port=2
  Add : Sum  Inputs=|+-
  PID Controller : slpidlib/PID Controller  Controller=PID  Form=Parallel  TimeDomain=Continuous-time  UseExternalTs=off  SampleTime=-1  IntegratorMethod=Forward Euler  FilterMethod=Forward Euler  ControllerParametersSource=internal  P=-2.16227850344127  I=-3.82729714855674  UseKiTs=off  D=-0.0839125504621507  UseExternalDerivativeSource=off  N=10.1322259704898  UseFilter=on  TunerSelectOption=Transfer Function Based (PID Tuner App)  InitialConditionSource=internal  InitialConditionForIntegrator=0  InitialConditionForFilter=0  DifferentiatorICPrevScaledInput=0  ExternalReset=none  TrackingMode=off  Kt=1  LimitOutput=off  SatLimitsSource=internal  UpperSaturationLimit=inf  LowerSaturationLimit=-inf  LinearizeAsGain=on  AntiWindupMode=none  Kb=1  LimitIntegrator=off  UpperIntegratorSaturationLimit=inf  LowerIntegratorSaturationLimit=-inf  POutMin=[]  POutMax=[]  IOutMin=[]  IOutMax=[]  DOutMin=[]  DOutMax=[]  NOutMin=[]  NOutMax=[]  SumOutMin=[]  SumOutMax=[]  SaturationOutMin=[]  SaturationOutMax=[]  PParamMin=[]  PParamMax=[]  IParamMin=[]  IParamMax=[]  DParamMin=[]  DParamMax=[]  NParamMin=[]  NParamMax=[]  KbParamMin=[]  KbParamMax=[]  KtParamMin=[]  KtParamMax=[]  KbOutMin=[]  KbOutMax=[]  KtOutMin=[]  KtOutMax=[]  IntegratorOutMin=[]  IntegratorOutMax=[]  FilterOutMin=[]  FilterOutMax=[]  SumI1OutMin=[]  SumI1OutMax=[]  SumI2OutMin=[]  SumI2OutMax=[]  SumI3OutMin=[]  SumI3OutMax=[]  SumI4OutMin=[]  SumI4OutMax=[]  SumDOutMin=[]  SumDOutMax=[]  DifferentiatorOutMin=[]  DifferentiatorOutMax=[]  FilterDiffOutCoefMin=[]  FilterDiffOutCoefMax=[]  ReciprocalOutMin=[]  ReciprocalOutMax=[]  SumDenOutMin=[]  SumDenOutMax=[]  SumNumOutMin=[]  SumNumOutMax=[]  DivideOutMin=[]  DivideOutMax=[]  UdiffTsProdOutMin=[]  UdiffTsProdOutMax=[]  NTsProdOutMin=[]  NTsProdOutMax=[]  UintegralTsProdOutMin=[]  UintegralTsProdOutMax=[]  UngainTsProdOutMin=[]  UngainTsProdOutMax=[]  ClampingZeroOutDataTypeStr=Inherit: Inherit via back propagation  ClampingZeroOutMin=[]  ClampingZeroOutMax=[]  FilterDenConstantOutDataTypeStr=Inherit: Inherit via back propagation  FilterDenConstantOutMin=[]  FilterDenConstantOutMax=[]  PCopyOutDataTypeStr=Inherit: Inherit via back propagation  PCopyOutMin=[]  PCopyOutMax=[]  NCopyOutDataTypeStr=Inherit: Inherit via back propagation  NCopyOutMin=[]  NCopyOutMax=[]  IntegratorContinuousStateAttributes=''  IntegratorStateMustResolveToSignalObject=off  IntegratorRTWStateStorageClass=Auto  FilterContinuousStateAttributes=''  FilterStateMustResolveToSignalObject=off  FilterRTWStateStorageClass=Auto  ParallelPVariant=InternalParameters  IdealPVariant=Disabled  IVariant=InternalParameters  DVariant=InternalParameters  IntegratorVariant=Continuous  SatVariant=Disabled  AWVariant=Passthrough  PCopyVariant=Disabled  TRVariant=Disabled  FdbkBlocksVariant=Forward  IdealPFdbkVariant=Disabled  SatFdbkVariant=Disabled  DerivativeFilterVariant=ContFilter  NVariant=InternalParameters  NCopyVariant=Disabled  FilterICVariant=InternalICsFilter  IntegratorICVariant=InternalICs  ExternalResetVariant=Disabled  TRSumVariant=Passthrough  SumFdbkVariant=Disabled  SumVariant=Sum_PID  TsampFilterVariant=InternalTs  TsampNgainVariant=Passthrough  TsampIntegralVariant=Disabled_SignalSpec  ExternalSaturationOutDataTypeStr=Inherit: Same as second input  DerivativeSourceVariant=ErrorSignal
  Y_cmd : Outport
  wires:
  Add/1 -> PID Controller/1  "psi_error"
  [Y_cmd] -> Y_cmd/1
  [psi_des] -> Add/1
  psi_des/1 -> [psi_des]
  PID Controller/1 -> [Y_cmd]
  psi_meas/1 -> [psi_meas]
  [psi_meas] -> Add/2

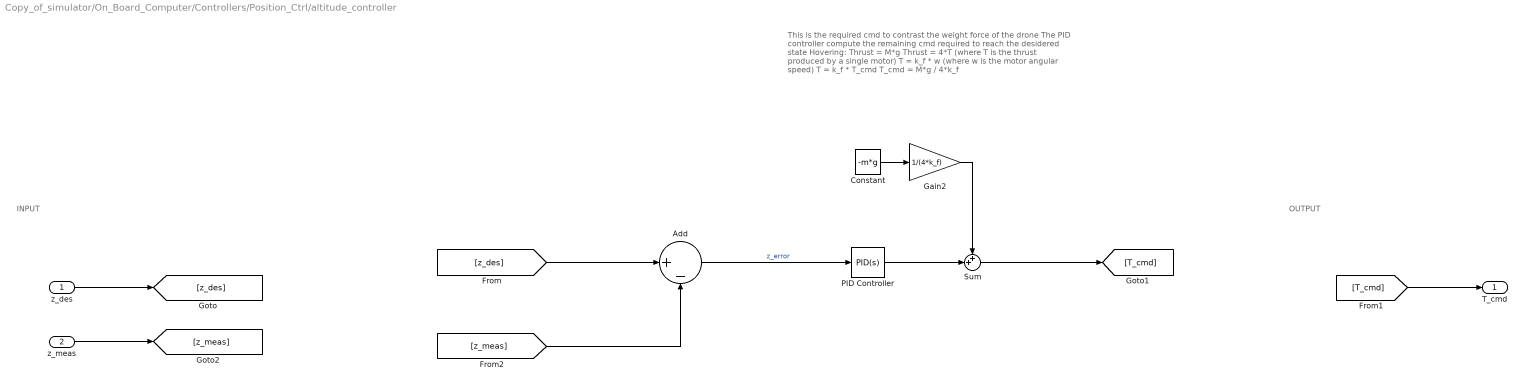
== system Copy_of_simulator/On_Board_Computer/Controllers/Position_Ctrl/altitude_controller ==
  note: OUTPUT
  note: INPUT
  note: This is the required cmd to contrast the weight force of the drone
      |
      | The PID controller compute the remaining cmd required to reach the
      | desidered state
      |
      | Hovering:
      | Thrust = M*g
      | Thrust = 4*T (where T is the thrust produced by a single motor)
      | T = k_f * w (where w is the motor angular speed)
      | T = k_f * T_cmd
      |
      | T_cmd = M*g / 4*k_f
  z_des : Inport
  z_meas : Inport  Port=2
  Add : Sum  Inputs=|+-
  Constant : Constant  Value=-m*g
  Gain2 : Gain  Gain=1/(4*k_f)
  PID Controller : slpidlib/PID Controller  Controller=PID  Form=Parallel  TimeDomain=Continuous-time  UseExternalTs=off  SampleTime=-1  IntegratorMethod=Forward Euler  FilterMethod=Forward Euler  ControllerParametersSource=internal  P=379867.55988404  I=17783.41559165  UseKiTs=off  D=1992473.36661034  UseExternalDerivativeSource=off  N=5.45397025421619  UseFilter=on  TunerSelectOption=Transfer Function Based (PID Tuner App)  InitialConditionSource=internal  InitialConditionForIntegrator=0  InitialConditionForFilter=0  DifferentiatorICPrevScaledInput=0  ExternalReset=none  TrackingMode=off  Kt=1  LimitOutput=off  SatLimitsSource=internal  UpperSaturationLimit=inf  LowerSaturationLimit=-inf  LinearizeAsGain=on  AntiWindupMode=none  Kb=1  LimitIntegrator=off  UpperIntegratorSaturationLimit=inf  LowerIntegratorSaturationLimit=-inf  POutMin=[]  POutMax=[]  IOutMin=[]  IOutMax=[]  DOutMin=[]  DOutMax=[]  NOutMin=[]  NOutMax=[]  SumOutMin=[]  SumOutMax=[]  SaturationOutMin=[]  SaturationOutMax=[]  PParamMin=[]  PParamMax=[]  IParamMin=[]  IParamMax=[]  DParamMin=[]  DParamMax=[]  NParamMin=[]  NParamMax=[]  KbParamMin=[]  KbParamMax=[]  KtParamMin=[]  KtParamMax=[]  KbOutMin=[]  KbOutMax=[]  KtOutMin=[]  KtOutMax=[]  IntegratorOutMin=[]  IntegratorOutMax=[]  FilterOutMin=[]  FilterOutMax=[]  SumI1OutMin=[]  SumI1OutMax=[]  SumI2OutMin=[]  SumI2OutMax=[]  SumI3OutMin=[]  SumI3OutMax=[]  SumI4OutMin=[]  SumI4OutMax=[]  SumDOutMin=[]  SumDOutMax=[]  DifferentiatorOutMin=[]  DifferentiatorOutMax=[]  FilterDiffOutCoefMin=[]  FilterDiffOutCoefMax=[]  ReciprocalOutMin=[]  ReciprocalOutMax=[]  SumDenOutMin=[]  SumDenOutMax=[]  SumNumOutMin=[]  SumNumOutMax=[]  DivideOutMin=[]  DivideOutMax=[]  UdiffTsProdOutMin=[]  UdiffTsProdOutMax=[]  NTsProdOutMin=[]  NTsProdOutMax=[]  UintegralTsProdOutMin=[]  UintegralTsProdOutMax=[]  UngainTsProdOutMin=[]  UngainTsProdOutMax=[]  ClampingZeroOutDataTypeStr=Inherit: Inherit via back propagation  ClampingZeroOutMin=[]  ClampingZeroOutMax=[]  FilterDenConstantOutDataTypeStr=Inherit: Inherit via back propagation  FilterDenConstantOutMin=[]  FilterDenConstantOutMax=[]  PCopyOutDataTypeStr=Inherit: Inherit via back propagation  PCopyOutMin=[]  PCopyOutMax=[]  NCopyOutDataTypeStr=Inherit: Inherit via back propagation  NCopyOutMin=[]  NCopyOutMax=[]  IntegratorContinuousStateAttributes=''  IntegratorStateMustResolveToSignalObject=off  IntegratorRTWStateStorageClass=Auto  FilterContinuousStateAttributes=''  FilterStateMustResolveToSignalObject=off  FilterRTWStateStorageClass=Auto  ParallelPVariant=InternalParameters  IdealPVariant=Disabled  IVariant=InternalParameters  DVariant=InternalParameters  IntegratorVariant=Continuous  SatVariant=Disabled  AWVariant=Passthrough  PCopyVariant=Disabled  TRVariant=Disabled  FdbkBlocksVariant=Forward  IdealPFdbkVariant=Disabled  SatFdbkVariant=Disabled  DerivativeFilterVariant=ContFilter  NVariant=InternalParameters  NCopyVariant=Disabled  FilterICVariant=InternalICsFilter  IntegratorICVariant=InternalICs  ExternalResetVariant=Disabled  TRSumVariant=Passthrough  SumFdbkVariant=Disabled  SumVariant=Sum_PID  TsampFilterVariant=InternalTs  TsampNgainVariant=Passthrough  TsampIntegralVariant=Disabled_SignalSpec  ExternalSaturationOutDataTypeStr=Inherit: Same as second input  DerivativeSourceVariant=ErrorSignal
  Sum : Sum  Inputs=++|
  T_cmd : Outport
  wires:
  [T_cmd] -> T_cmd/1
  z_des/1 -> [z_des]
  z_meas/1 -> [z_meas]
  Add/1 -> PID Controller/1  "z_error"
  [z_des] -> Add/1
  PID Controller/1 -> Sum/2
  [z_meas] -> Add/2
  Constant/1 -> Gain2/1
  Sum/1 -> [T_cmd]
  Gain2/1 -> Sum/1

== system Copy_of_simulator/On_Board_Computer/Controllers/Position_Ctrl/phi_controller ==
  note: OUTPUT
  note: INPUT
  y_des : Inport
  y_meas : Inport  Port=2
  Add : Sum  Inputs=|+-
  PID Controller : slpidlib/PID Controller  Controller=PID  Form=Parallel  TimeDomain=Continuous-time  UseExternalTs=off  SampleTime=-1  IntegratorMethod=Forward Euler  FilterMethod=Forward Euler  ControllerParametersSource=internal  P=100  I=200  UseKiTs=off  D=50  UseExternalDerivativeSource=off  N=10.1322259704898  UseFilter=on  TunerSelectOption=Transfer Function Based (PID Tuner App)  InitialConditionSource=internal  InitialConditionForIntegrator=0  InitialConditionForFilter=0  DifferentiatorICPrevScaledInput=0  ExternalReset=none  TrackingMode=off  Kt=1  LimitOutput=off  SatLimitsSource=internal  UpperSaturationLimit=inf  LowerSaturationLimit=-inf  LinearizeAsGain=on  AntiWindupMode=none  Kb=1  LimitIntegrator=off  UpperIntegratorSaturationLimit=inf  LowerIntegratorSaturationLimit=-inf  POutMin=[]  POutMax=[]  IOutMin=[]  IOutMax=[]  DOutMin=[]  DOutMax=[]  NOutMin=[]  NOutMax=[]  SumOutMin=[]  SumOutMax=[]  SaturationOutMin=[]  SaturationOutMax=[]  PParamMin=[]  PParamMax=[]  IParamMin=[]  IParamMax=[]  DParamMin=[]  DParamMax=[]  NParamMin=[]  NParamMax=[]  KbParamMin=[]  KbParamMax=[]  KtParamMin=[]  KtParamMax=[]  KbOutMin=[]  KbOutMax=[]  KtOutMin=[]  KtOutMax=[]  IntegratorOutMin=[]  IntegratorOutMax=[]  FilterOutMin=[]  FilterOutMax=[]  SumI1OutMin=[]  SumI1OutMax=[]  SumI2OutMin=[]  SumI2OutMax=[]  SumI3OutMin=[]  SumI3OutMax=[]  SumI4OutMin=[]  SumI4OutMax=[]  SumDOutMin=[]  SumDOutMax=[]  DifferentiatorOutMin=[]  DifferentiatorOutMax=[]  FilterDiffOutCoefMin=[]  FilterDiffOutCoefMax=[]  ReciprocalOutMin=[]  ReciprocalOutMax=[]  SumDenOutMin=[]  SumDenOutMax=[]  SumNumOutMin=[]  SumNumOutMax=[]  DivideOutMin=[]  DivideOutMax=[]  UdiffTsProdOutMin=[]  UdiffTsProdOutMax=[]  NTsProdOutMin=[]  NTsProdOutMax=[]  UintegralTsProdOutMin=[]  UintegralTsProdOutMax=[]  UngainTsProdOutMin=[]  UngainTsProdOutMax=[]  ClampingZeroOutDataTypeStr=Inherit: Inherit via back propagation  ClampingZeroOutMin=[]  ClampingZeroOutMax=[]  FilterDenConstantOutDataTypeStr=Inherit: Inherit via back propagation  FilterDenConstantOutMin=[]  FilterDenConstantOutMax=[]  PCopyOutDataTypeStr=Inherit: Inherit via back propagation  PCopyOutMin=[]  PCopyOutMax=[]  NCopyOutDataTypeStr=Inherit: Inherit via back propagation  NCopyOutMin=[]  NCopyOutMax=[]  IntegratorContinuousStateAttributes=''  IntegratorStateMustResolveToSignalObject=off  IntegratorRTWStateStorageClass=Auto  FilterContinuousStateAttributes=''  FilterStateMustResolveToSignalObject=off  FilterRTWStateStorageClass=Auto  ParallelPVariant=InternalParameters  IdealPVariant=Disabled  IVariant=InternalParameters  DVariant=InternalParameters  IntegratorVariant=Continuous  SatVariant=Disabled  AWVariant=Passthrough  PCopyVariant=Disabled  TRVariant=Disabled  FdbkBlocksVariant=Forward  IdealPFdbkVariant=Disabled  SatFdbkVariant=Disabled  DerivativeFilterVariant=ContFilter  NVariant=InternalParameters  NCopyVariant=Disabled  FilterICVariant=InternalICsFilter  IntegratorICVariant=InternalICs  ExternalResetVariant=Disabled  TRSumVariant=Passthrough  SumFdbkVariant=Disabled  SumVariant=Sum_PID  TsampFilterVariant=InternalTs  TsampNgainVariant=Passthrough  TsampIntegralVariant=Disabled_SignalSpec  ExternalSaturationOutDataTypeStr=Inherit: Same as second input  DerivativeSourceVariant=ErrorSignal
  phi_des : Outport
  wires:
  Add/1 -> PID Controller/1  "y_error"
  [phi_des] -> phi_des/1
  [y_des] -> Add/1
  y_des/1 -> [y_des]
  PID Controller/1 -> [phi_des]
  y_meas/1 -> [y_meas]
  [y_meas] -> Add/2

== system Copy_of_simulator/On_Board_Computer/Controllers/Position_Ctrl/theta_controller ==
  note: OUTPUT
  note: INPUT
  x_des : Inport
  x_meas : Inport  Port=2
  Add : Sum  Inputs=|+-
  PID Controller : slpidlib/PID Controller  Controller=PID  Form=Parallel  TimeDomain=Continuous-time  UseExternalTs=off  SampleTime=-1  IntegratorMethod=Forward Euler  FilterMethod=Forward Euler  ControllerParametersSource=internal  P=-0.597169985490015  I=-1.05700860413316  UseKiTs=off  D=-0.0231746541725141  UseExternalDerivativeSource=off  N=10.1322259704898  UseFilter=on  TunerSelectOption=Transfer Function Based (PID Tuner App)  InitialConditionSource=internal  InitialConditionForIntegrator=0  InitialConditionForFilter=0  DifferentiatorICPrevScaledInput=0  ExternalReset=none  TrackingMode=off  Kt=1  LimitOutput=off  SatLimitsSource=internal  UpperSaturationLimit=inf  LowerSaturationLimit=-inf  LinearizeAsGain=on  AntiWindupMode=none  Kb=1  LimitIntegrator=off  UpperIntegratorSaturationLimit=inf  LowerIntegratorSaturationLimit=-inf  POutMin=[]  POutMax=[]  IOutMin=[]  IOutMax=[]  DOutMin=[]  DOutMax=[]  NOutMin=[]  NOutMax=[]  SumOutMin=[]  SumOutMax=[]  SaturationOutMin=[]  SaturationOutMax=[]  PParamMin=[]  PParamMax=[]  IParamMin=[]  IParamMax=[]  DParamMin=[]  DParamMax=[]  NParamMin=[]  NParamMax=[]  KbParamMin=[]  KbParamMax=[]  KtParamMin=[]  KtParamMax=[]  KbOutMin=[]  KbOutMax=[]  KtOutMin=[]  KtOutMax=[]  IntegratorOutMin=[]  IntegratorOutMax=[]  FilterOutMin=[]  FilterOutMax=[]  SumI1OutMin=[]  SumI1OutMax=[]  SumI2OutMin=[]  SumI2OutMax=[]  SumI3OutMin=[]  SumI3OutMax=[]  SumI4OutMin=[]  SumI4OutMax=[]  SumDOutMin=[]  SumDOutMax=[]  DifferentiatorOutMin=[]  DifferentiatorOutMax=[]  FilterDiffOutCoefMin=[]  FilterDiffOutCoefMax=[]  ReciprocalOutMin=[]  ReciprocalOutMax=[]  SumDenOutMin=[]  SumDenOutMax=[]  SumNumOutMin=[]  SumNumOutMax=[]  DivideOutMin=[]  DivideOutMax=[]  UdiffTsProdOutMin=[]  UdiffTsProdOutMax=[]  NTsProdOutMin=[]  NTsProdOutMax=[]  UintegralTsProdOutMin=[]  UintegralTsProdOutMax=[]  UngainTsProdOutMin=[]  UngainTsProdOutMax=[]  ClampingZeroOutDataTypeStr=Inherit: Inherit via back propagation  ClampingZeroOutMin=[]  ClampingZeroOutMax=[]  FilterDenConstantOutDataTypeStr=Inherit: Inherit via back propagation  FilterDenConstantOutMin=[]  FilterDenConstantOutMax=[]  PCopyOutDataTypeStr=Inherit: Inherit via back propagation  PCopyOutMin=[]  PCopyOutMax=[]  NCopyOutDataTypeStr=Inherit: Inherit via back propagation  NCopyOutMin=[]  NCopyOutMax=[]  IntegratorContinuousStateAttributes=''  IntegratorStateMustResolveToSignalObject=off  IntegratorRTWStateStorageClass=Auto  FilterContinuousStateAttributes=''  FilterStateMustResolveToSignalObject=off  FilterRTWStateStorageClass=Auto  ParallelPVariant=InternalParameters  IdealPVariant=Disabled  IVariant=InternalParameters  DVariant=InternalParameters  IntegratorVariant=Continuous  SatVariant=Disabled  AWVariant=Passthrough  PCopyVariant=Disabled  TRVariant=Disabled  FdbkBlocksVariant=Forward  IdealPFdbkVariant=Disabled  SatFdbkVariant=Disabled  DerivativeFilterVariant=ContFilter  NVariant=InternalParameters  NCopyVariant=Disabled  FilterICVariant=InternalICsFilter  IntegratorICVariant=InternalICs  ExternalResetVariant=Disabled  TRSumVariant=Passthrough  SumFdbkVariant=Disabled  SumVariant=Sum_PID  TsampFilterVariant=InternalTs  TsampNgainVariant=Passthrough  TsampIntegralVariant=Disabled_SignalSpec  ExternalSaturationOutDataTypeStr=Inherit: Same as second input  DerivativeSourceVariant=ErrorSignal
  theta_des : Outport
  wires:
  x_des/1 -> [x_des]
  [x_des] -> Add/1
  [theta_des] -> theta_des/1
  x_meas/1 -> [x_meas]
  [x_meas] -> Add/2
  Add/1 -> PID Controller/1  "x_error"
  PID Controller/1 -> [theta_des]
